simulink library "visualservolib"  (R2023a)
settings: Solver=VariableStepAuto  StartTime=0.0  StopTime=10.0  RelTol=1e-3
values from neighbouring files (symbols this model uses):
  D = diag( g.connectivity() )    [PGraph.m]    (also in UGraph.m)
undefined symbols (not defined in the file or in its folder): camera, cond, delta2tform, tformnorm, tformrz
Description:
  | Simulink library with commonly used blocks for
  | Robotics, Vision and Control - 3rd Edition
settings Model: Creator=rpill  LastModifiedBy=rpill
settings SolverCC: MaxZcPerStep=1
settings DebuggingCC: UnconnectedInputMsg=warning  UnconnectedOutputMsg=warning  UnconnectedLineMsg=warning
settings ModelReferenceCC: EnableRefExpFcnMdlSchedulingChecks=on
settings RTWCC: DLArmComputeVersion=19.05

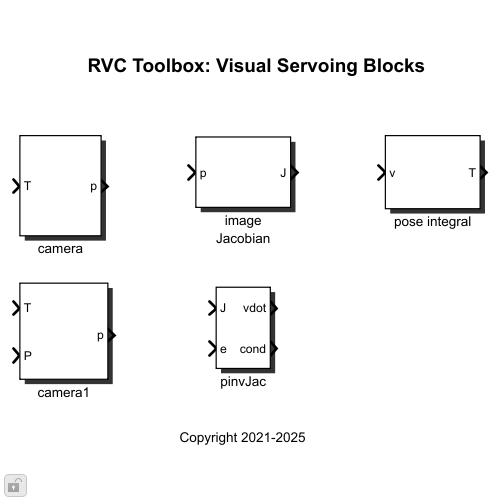
[thumbnail: Simulink's stored preview of the top-level diagram]
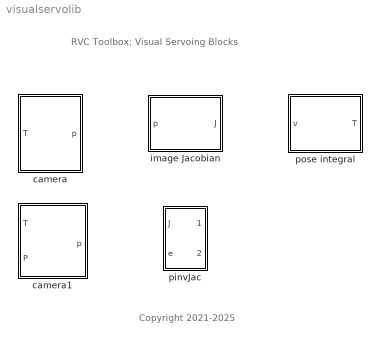
== system visualservolib ==
  note: Copyright 2021-2025
  note: RVC Toolbox: Visual Servoing Blocks
  camera : Subsystem  mask{cam=[], points=[]}
      mask prompts: cam "Camera"; points "Points (3xN)"
      mask help: Camera model
      mask Help:
      | A generalized camera model that projects a set of world points to the image
      | plane.
      | 
      | 
      | <b>Parameters::</b>
      | 
      | Camera (Camera)  The camera object, subclass of Camera class
      | Points (3xN)     The 3D world points, one per column
      | 
      | <b>Inputs::</b>
      | 
      | T (4x4) the camera pose as a homogeneous transformation
      | 
      | 
      | <b>Outputs::</b>
      | 
      | p (2xN) projection of world points, one per column, corresponding to columns
      |         of the parameter Points.
      | 
      | <b>Notes::</b>
      | 
      | - Accepts any camera object derived from the abstract Camera superclass.
  camera1 : Subsystem  mask{cam=camera}
      mask prompts: cam "Camera"
      mask help: Camera model for moving object
      mask Help:
      | A generalized camera model that projects a set of world points to the image
      | plane.
      | 
      | 
      | <b>Parameters::</b>
      | 
      | Camera (Camera)  The camera object, subclass of Camera class
      | Points (3xN)     The 3D world points, one per column, with respect to the
      |                  object coordinate frame.
      | 
      | <b>Inputs::</b>
      | 
      | T (4x4)    the camera pose as a homogeneous transformation
      | Tobj (4x4) the pose of the object coordinate frame
      | 
      | <b>Outputs::</b>
      | 
      | p (2xN) projection of world points, one per column, corresponding to columns
      |         of the parameter Points.
      | 
      | <b>Notes::</b>
      | 
      | - This block allows for the object to move, as well as the camera.
      | - Accepts any camera object derived from the abstract Camera superclass.
  image Jacobian : Subsystem  mask{cam=camera, z=1}
      mask prompts: cam "Camera"; z "Assumed depth (m)"
      mask help: Image Jacobian
      mask Help:
      | Jacobian matrix relating image plane point velocity to camera spatial
      | velocity expressed in the world frame.
      | 
      | <b>Parameters::</b>
      | 
      | Camera (Camera)  The camera object, subclass of Camera class
      | z (1x1)          Point depth, assumed same for all points
      | z (1xN)          Point depth, unique for each point
      | 
      | <b>Inputs::</b>
      | 
      | Points (2xN)     The 2D image-plane points, one per column
      | 
      | 
      | <b>Outputs::</b>
      | 
      | J (2Nx6) the image Jacobian matrix
      | 
      | <b>Notes::</b>
      | 
      | - For multiple points the Jacobian is the "stack" of the 2x6 point feature
      |   Jacobians.
      | - A wrapper for the Toolbox method visjac_p().
  pinvJac : Subsystem
      mask help: Inverse image Jacobian
      mask Help:
      | Computes camera velocity based on the pseudo-inverse of the image Jacobian
      | and image plane error for more than 3 points.
      | 
      | 
      | <b>Inputs::</b>
      | 
      | J (2Nx6) the image Jacobian matrix
      | e (2Nx1) the image plane error (du1, dv1, du2, dv2, ...)
      | 
      | <b>Outputs::</b>
      | 
      | vdot (1x6) the required camera spatial velocity
      | cond (1x1) the condition of the image Jacobian
      | 
      | <b>Notes::</b>
      | 
      | - A wrapper for the MATLAB function pinv().
      | - Valid for non-square Jacobians (>=3 image points)
  pose integral : Subsystem  mask{T0=tformrz(1.5), dt=0.02}
      mask prompts: T0 "Initial pose (hom transform)"; dt "Sample interval (s)"
      mask help: Integrate spatial velocity
      mask Help:
      | Integrate spatial velocity to update pose represented as a homogeneous
      | transformation.
      | 
      | <b>Parameters::</b>
      | 
      | T0 (4x4)  The initial pose
      | dt (1x1)  The sample interval [s]
      | 
      | <b>Inputs::</b>
      | 
      | v (1x6) spatial velocity (xd yd zd wx wy wz)
      | 
      | <b>Outputs::</b>
      | 
      | T (4x4) the integrated pose as a homogeneous transformation
      | 
      | <b>Notes::</b>
      | 
      | - Contains a unit delay of dt
      | - The transform is kept normalized using trnorm().

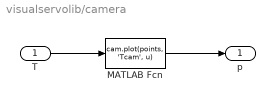
== system visualservolib/camera ==
  T : Inport
  MATLAB Fcn : MATLABFcn  MATLABFcn=cam.plot(points, 'Tcam', u)  OutputSignalType=real  Output1D=off
  p : Outport  VectorParamsAs1DForOutWhenUnconnected=off
  wires:
  MATLAB Fcn/1 -> p/1
  T/1 -> MATLAB Fcn/1

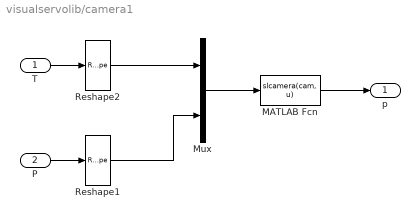
== system visualservolib/camera1 ==
  T : Inport
  P : Inport  Port=2
  MATLAB Fcn : MATLABFcn  MATLABFcn=slcamera(cam, u)  OutputSignalType=real  Output1D=off
  Mux : Mux  Inputs=2
  Reshape1 : Reshape  OutputDimensionality=Column vector (2-D)  OutputDimensions=6
  Reshape2 : Reshape  OutputDimensionality=Column vector (2-D)  OutputDimensions=6
  p : Outport  VectorParamsAs1DForOutWhenUnconnected=off
  wires:
  Reshape1/1 -> Mux/2
  Reshape2/1 -> Mux/1
  P/1 -> Reshape1/1
  T/1 -> Reshape2/1
  Mux/1 -> MATLAB Fcn/1
  MATLAB Fcn/1 -> p/1

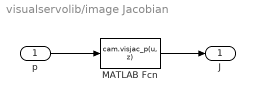
== system visualservolib/image Jacobian ==
  p : Inport
  MATLAB Fcn : MATLABFcn  MATLABFcn=cam.visjac_p(u, z)  Output1D=off
  J : Outport  VectorParamsAs1DForOutWhenUnconnected=off
  wires:
  MATLAB Fcn/1 -> J/1
  p/1 -> MATLAB Fcn/1

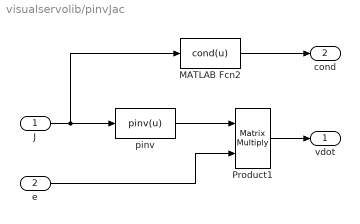
== system visualservolib/pinvJac ==
  J : Inport
  e : Inport  Port=2
  MATLAB Fcn2 : MATLABFcn  MATLABFcn=cond(u)  Output1D=off
  Product1 : Product  Multiplication=Matrix(*)  InputSameDT=on  RndMeth=Zero  SaturateOnIntegerOverflow=on  OutDataTypeStr=Inherit: Same as first input
  pinv : MATLABFcn  MATLABFcn=pinv(u)  Output1D=off
  vdot : Outport  VectorParamsAs1DForOutWhenUnconnected=off
  cond : Outport  Port=2  VectorParamsAs1DForOutWhenUnconnected=off
  wires:
  J/1 -> MATLAB Fcn2/1, pinv/1
  pinv/1 -> Product1/1
  e/1 -> Product1/2
  MATLAB Fcn2/1 -> cond/1
  Product1/1 -> vdot/1

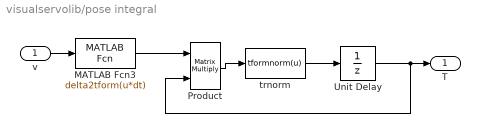
== system visualservolib/pose integral ==
  v : Inport
  MATLAB Fcn3 : MATLABFcn  MATLABFcn=delta2tform(u*dt)  OutputDimensions=[4,4]  Output1D=off
  Product : Product  Multiplication=Matrix(*)  RndMeth=Zero
  Unit Delay : UnitDelay  InitialCondition=T0  SampleTime=dt  HasFrameUpgradeWarning=on
  trnorm : MATLABFcn  MATLABFcn=tformnorm(u)  Output1D=off
  T : Outport  VectorParamsAs1DForOutWhenUnconnected=off
  wires:
  v/1 -> MATLAB Fcn3/1
  trnorm/1 -> Unit Delay/1
  MATLAB Fcn3/1 -> Product/1
  Unit Delay/1 -> T/1, Product/2
  Product/1 -> trnorm/1
